simulink model "simulink_Qdot"  (R2022b)
settings: Solver=FixedStepAuto  StartTime=0.0  StopTime=10.0  FixedStep=0.1  RelTol=1e-3
settings Model: Creator=Ziad  LastModifiedBy=Ziad

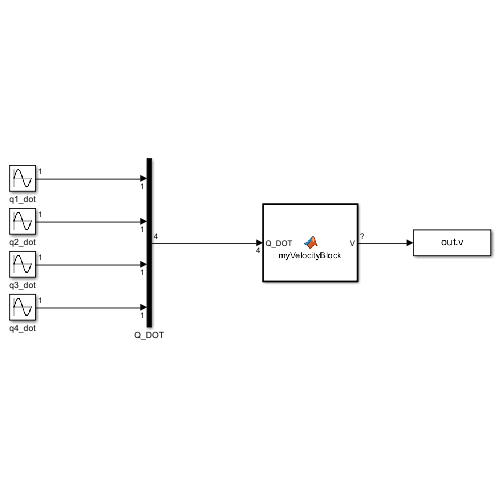
[thumbnail: Simulink's stored preview of the top-level diagram]
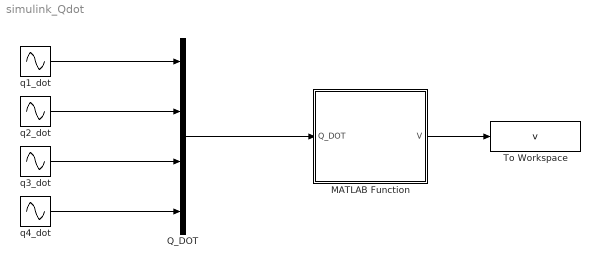
== system simulink_Qdot ==
  MATLAB Function : MATLAB Function  TreatAsAtomicUnit=on
  Q_DOT : Mux
  To Workspace : ToWorkspace  VariableName=v  SampleTime=-1
      settings: Save2DSignal=2-D array (concatenate along first dimension)
  q1_dot : Sin  SampleTime=0
  q2_dot : Sin  SampleTime=0
  q3_dot : Sin  SampleTime=0
  q4_dot : Sin  SampleTime=0
  wires:
  q1_dot/1 -> Q_DOT/1
  q2_dot/1 -> Q_DOT/2
  q3_dot/1 -> Q_DOT/3
  q4_dot/1 -> Q_DOT/4
  Q_DOT/1 -> MATLAB Function/1(Q_DOT)
  MATLAB Function/1(V) -> To Workspace/1

== matlab function simulink_Qdot/MATLAB Function ==
  data: Q_DOT input; V output

function V = myVelocityBlock(Q_DOT)
    coder.extrinsic('syms');
    coder.extrinsic('myVelocityBlock');
    V = Velocity_kinematics(Q_DOT);
    
end
